simulink model "System_model"  (R2023b)
settings: Solver=VariableStepAuto  StartTime=0.0  StopTime=120  RelTol=1e-3
libraries: dspmathops x5, dspstat3 x4, audiodynamicrange x2, audiofilters x2, audiosources x1, simulink x1
settings Model: Creator=Khash  LastModifiedBy=Khash

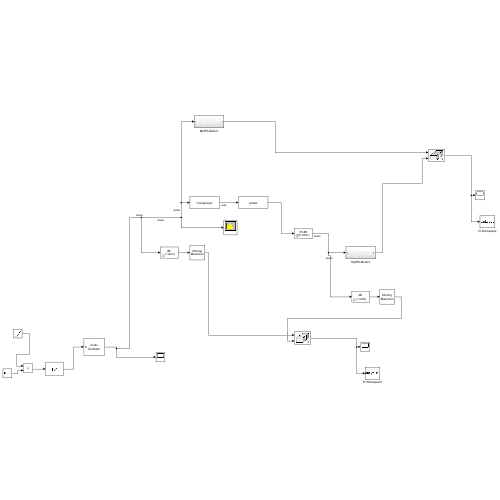
[thumbnail: Simulink's stored preview of the top-level diagram]
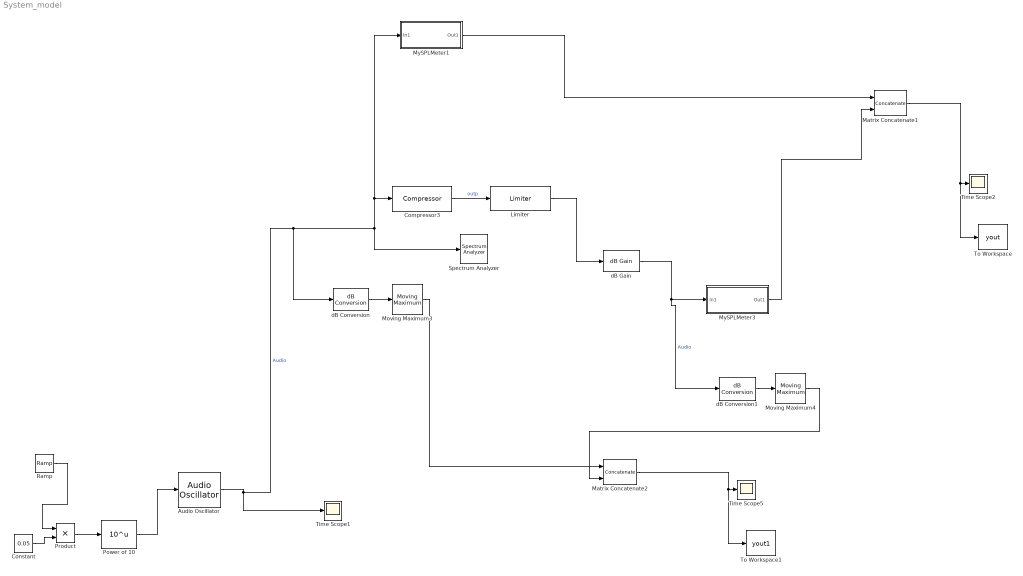
== system System_model ==
  Audio Oscillator : audiosources/Audio Oscillator  FrequencyPort=off  Frequency=1000  AmplitudePort=on  Amplitude=10  DCOffsetPort=off  PhaseOffset=0  DCOffset=0  WidthPort=off  Width=1  DutyCyclePort=off  DutyCycle=0.5  SampsPerFrame=512  Fs=44100  OutputDataType=double  SimulateUsing=Code generation
      settings: SignalType=sine
  Compressor3 : audiodynamicrange/Compressor  ThresholdPort=off  Threshold=-50  RatioPort=off  Ratio=2  KneeWidthPort=off  KneeWidth=0.0  AttackTimePort=off  AttackTime=0  ReleaseTimePort=off  ReleaseTime=0.0  MakeUpGainMode=Property  MakeUpGain=0.0  InheritSampleRate=off  SampleRate=44100  outputGain=off  EnableSidechain=off  SimulateUsing=Code generation
  Constant : Constant  Value=0.05
  Limiter : audiodynamicrange/Limiter  ThresholdPort=off  Threshold=-20  KneeWidthPort=off  KneeWidth=0.0  AttackTimePort=off  AttackTime=0.0  ReleaseTimePort=off  ReleaseTime=0  MakeUpGainMode=Property  MakeUpGain=0.0  InheritSampleRate=off  SampleRate=44100  outputGain=off  EnableSidechain=off  SimulateUsing=Code generation
  Matrix Concatenate1 : Concatenate  Mode=Multidimensional array  ConcatenateDimension=2
  Matrix Concatenate2 : Concatenate  Mode=Multidimensional array  ConcatenateDimension=2
  Moving Maximum3 : dspstat3/Moving Maximum  SpecifyWindowLength=on  WindowLength=44100  SimulateUsing=Code generation
  Moving Maximum4 : dspstat3/Moving Maximum  SpecifyWindowLength=on  WindowLength=44100  SimulateUsing=Code generation
  MySPLMeter1 : Subsystem
  MySPLMeter3 : Subsystem
  Power of 10 : Math  Operator=10^u
  Product : Product
  Ramp : simulink/Sources/Ramp  slope=1  start=0  InitialOutput=-90
  Spectrum Analyzer : SpectrumAnalyzer  WindowPosition=[239.000000,229.000000,800.000000,500.000000,]  Visible=on  ScopeFrameLocation=window  SampleRateSource=Property  SampleRate=44.1e3  PlotAsTwoSidedSpectrum=off  FrequencyScale=Log  FrequencySpan=Start and stop frequencies  StartFrequency=20  StopFrequency=20e3  YLimits=[-239.40180872,88.91711446]  SelectedToolstripTab=spectrumAnalyzerToolstrip.spectrumTab
  Time Scope1 : Scope
  Time Scope2 : Scope
  Time Scope5 : Scope
  To Workspace : ToWorkspace  VariableName=yout  SampleTime=-1
      settings: Save2DSignal=2-D array (concatenate along first dimension)
  To Workspace1 : ToWorkspace  VariableName=yout1  SampleTime=-1
      settings: Save2DSignal=2-D array (concatenate along first dimension)
  dB Conversion : dspmathops/dB Conversion  dBtype=dB  intype=Amplitude  R=1  fuzz=off
  dB Conversion1 : dspmathops/dB Conversion  dBtype=dB  intype=Amplitude  R=1  fuzz=off
  dB Gain : dspmathops/dB Gain  dB=35  intype=Amplitude
  wires:
  Matrix Concatenate1/1 -> To Workspace/1, Time Scope2/1
  Compressor3/1 -> Limiter/1  "outp"
  dB Conversion/1 -> Moving Maximum3/1
  dB Conversion1/1 -> Moving Maximum4/1
  dB Gain/1 -> dB Conversion1/1, MySPLMeter3/1(In1)  "Audio"
  Moving Maximum4/1 -> Matrix Concatenate2/2
  Moving Maximum3/1 -> Matrix Concatenate2/1
  Matrix Concatenate2/1 -> To Workspace1/1, Time Scope5/1
  Audio Oscillator/1 -> Time Scope1/1, dB Conversion/1, MySPLMeter1/1(In1), Compressor3/1, Spectrum Analyzer/1  "Audio"
  Limiter/1 -> dB Gain/1
  MySPLMeter1/1(Out1) -> Matrix Concatenate1/1
  MySPLMeter3/1(Out1) -> Matrix Concatenate1/2
  Product/1 -> Power of 10/1
  Power of 10/1 -> Audio Oscillator/1
  Ramp/1 -> Product/1
  Constant/1 -> Product/2

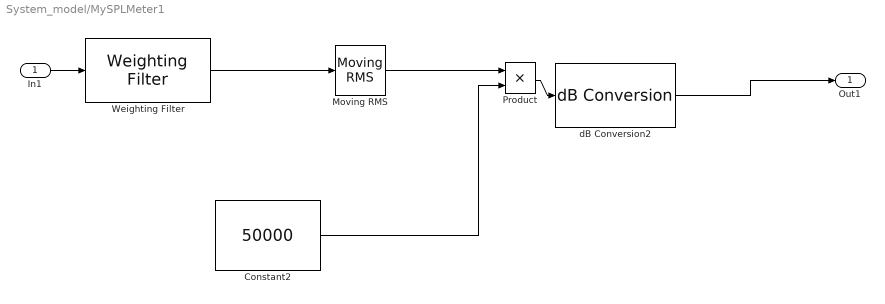
== system System_model/MySPLMeter1 ==
  In1 : Inport
  Constant2 : Constant  Value=50000
  Moving RMS : dspstat3/Moving RMS  Method=Sliding window  ForgettingFactorPort=off  SpecifyWindowLength=on  WindowLength=44100  OverlapLength=44099  AllowArbitraryInputLength=off  ForgettingFactor=0.9  SimulateUsing=Code generation
  Product : Product
  Weighting Filter : audiofilters/Weighting Filter  Method=A-weighting  InheritSampleRate=off  SampleRate=44100  SimulateUsing=Code generation  WorkspaceVariableName=myFilt  OverwriteExportVariable=on  MaskClassType=No mask
  dB Conversion2 : dspmathops/dB Conversion  dBtype=dB  intype=Amplitude  R=1  fuzz=off
  Out1 : Outport
  wires:
  dB Conversion2/1 -> Out1/1
  Constant2/1 -> Product/2
  Product/1 -> dB Conversion2/1
  In1/1 -> Weighting Filter/1
  Weighting Filter/1 -> Moving RMS/1
  Moving RMS/1 -> Product/1

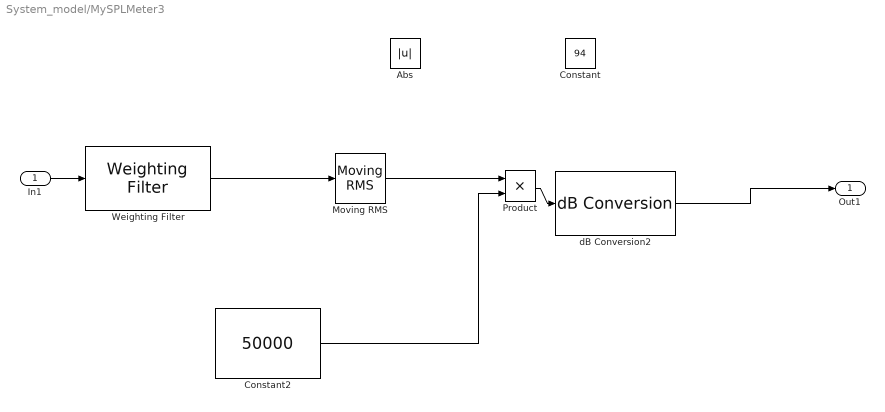
== system System_model/MySPLMeter3 ==
  In1 : Inport
  Abs : Abs  SaturateOnIntegerOverflow=off
  Constant : Constant  Value=94
  Constant2 : Constant  Value=50000
  Moving RMS : dspstat3/Moving RMS  Method=Sliding window  ForgettingFactorPort=off  SpecifyWindowLength=on  WindowLength=44100  OverlapLength=44099  AllowArbitraryInputLength=off  ForgettingFactor=0.9  SimulateUsing=Code generation
  Product : Product
  Weighting Filter : audiofilters/Weighting Filter  Method=A-weighting  InheritSampleRate=off  SampleRate=44100  SimulateUsing=Code generation  WorkspaceVariableName=myFilt  OverwriteExportVariable=on  MaskClassType=No mask
  dB Conversion2 : dspmathops/dB Conversion  dBtype=dB  intype=Amplitude  R=1  fuzz=off
  Out1 : Outport
  wires:
  dB Conversion2/1 -> Out1/1
  Constant2/1 -> Product/2
  Product/1 -> dB Conversion2/1
  In1/1 -> Weighting Filter/1
  Weighting Filter/1 -> Moving RMS/1
  Moving RMS/1 -> Product/1
